simulink model "logistic_growth"  (R2023b)
settings: Solver=FixedStepAuto  StartTime=0.0  StopTime=500  FixedStep=0.01  RelTol=1e-3
settings Model: Creator=vaclav  LastModifiedBy=vaclav
settings OptimizationCC: ReuseModelBlockBuffer=off

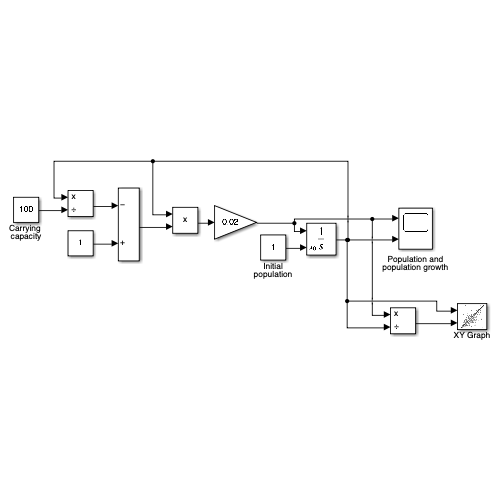
[thumbnail: Simulink's stored preview of the top-level diagram]
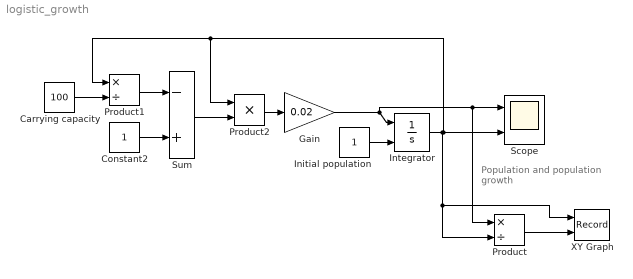
== system logistic_growth ==
  note: Population and
      | population growth
  Carrying capacity : Constant  Value=100
  Constant2 : Constant
  Gain : Gain  Gain=0.02
  Initial population : Constant
  Integrator : Integrator  InitialConditionSource=external
  Product : Product  Inputs=*/
  Product1 : Product  Inputs=*/
  Product2 : Product
  Scope : Scope  NumInputPorts=2
  Sum : Sum  Inputs=-+
  XY Graph : Record  FileSettingsInternal="{\"entries\":[{\"content\":{\"excelSettings\":{\"content\":{},\"type\":\"Streamout.ExcelSettings\"}},\"type\":\"Streamout.FileSettingStorage\",\"uuid\":\"\"}],\"packageUris\":[\"http:\\/\\/schema.mathworks.com\\/mf0\\/streamout_blocks\\/R2020a\"],\"version\":\"1.0\"}"  Layout=[1 1]  SignalsInternal="{\"entries\":[{\"content\":{\"signals\":[{\"content\":{\"blockPath\":[],\"dimensions\":[1],\"domain\":\"\",\"lineColor\":\"#a2142f\",\"plots\":[ 1 ],\"port\":1,\"sid\":[\"\"],\"signalID\":1,\"signalName\":\"Integrator\"},\"type\":\"RecordBlkView.Signal\",\"uuid\":\"\"},{\"content\":{\"blockPath\":[],\"dimensions\":[1],\"domain\":\"\",\"lineColor\":\"#139fff\",\"plots\":[ 1 ],\"port\":2,\"sid\":[\"\"],\"signalID\":2,\"signalName\":\"Product\"},\"type\":\"RecordBlkView.Signal\",\"uuid\":\"\"}]},\"type\":\"RecordBlkView.InputSignals\",\"uuid\":\"\"}],\"packageUris\":[\"http:\\/\\/schema.mathworks.com\\/mf0\\/streamout_blocks\\/R2020a\"],\"version\":\"1.0\"}"  VisualizationBindings="{\"xyplotplugin\":{\"info\":[{\"series\":[{\"bindingParametersList\":[{\"parameter\":\"X-Axis\",\"signalID\":1,\"signalName\":\"Integrator\"},{\"parameter\":\"Y-Axis\",\"signalID\":2,\"signalName\":\"Product\"}],\"seriesID\":0}],\"subplotID\":1}]}}"  CompatibilityTag=XY
  wires:
  Product2/1 -> Gain/1
  Integrator/1 -> Product1/1, Product2/1, Scope/2, Product/2, XY Graph/1
  Initial population/1 -> Integrator/2
  Sum/1 -> Product2/2
  Carrying capacity/1 -> Product1/2
  Constant2/1 -> Sum/2
  Product1/1 -> Sum/1
  Product/1 -> XY Graph/2
  Gain/1 -> Integrator/1, Product/1, Scope/1
